simulink model "questa6_trab1"  (R2020a)
settings: Solver=VariableStepAuto  StartTime=0.0  StopTime=10  RelTol=1e-3
settings Model: Creator=luang  LastModifiedBy=lafai

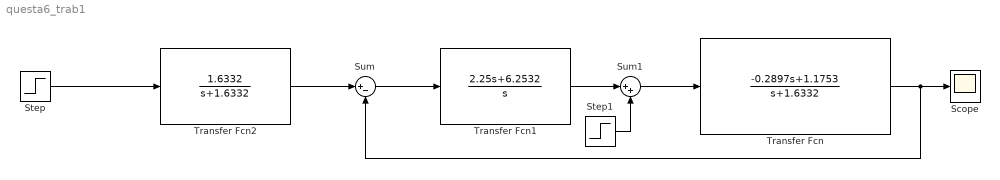
== system questa6_trab1 ==
  Scope : Scope
  Step : Step  Time=0  SampleTime=0
  Step1 : Step  Time=5  SampleTime=0
  Sum : Sum  Inputs=|+-
  Sum1 : Sum  Inputs=|++
  Transfer Fcn : TransferFcn  Numerator=[-0.2897 1.1753]  Denominator=[1 1.6332]
  Transfer Fcn1 : TransferFcn  Numerator=[2.25 6.2532]  Denominator=[1 0]
  Transfer Fcn2 : TransferFcn  Numerator=[1.6332]  Denominator=[1 1.6332]
  wires:
  Sum/1 -> Transfer Fcn1/1
  Transfer Fcn/1 -> Sum/2, Scope/1
  Transfer Fcn2/1 -> Sum/1
  Step/1 -> Transfer Fcn2/1
  Transfer Fcn1/1 -> Sum1/1
  Sum1/1 -> Transfer Fcn/1
  Step1/1 -> Sum1/2
